simulink model "Pitch_control_v5_test_english"  (R2017b)
settings: Solver=VariableStepAuto  StartTime=0.0  StopTime=60  MaxStep=0.01  RelTol=1e-3
libraries: simulink x2
settings Model: Creator=robo  LastModifiedBy=ad

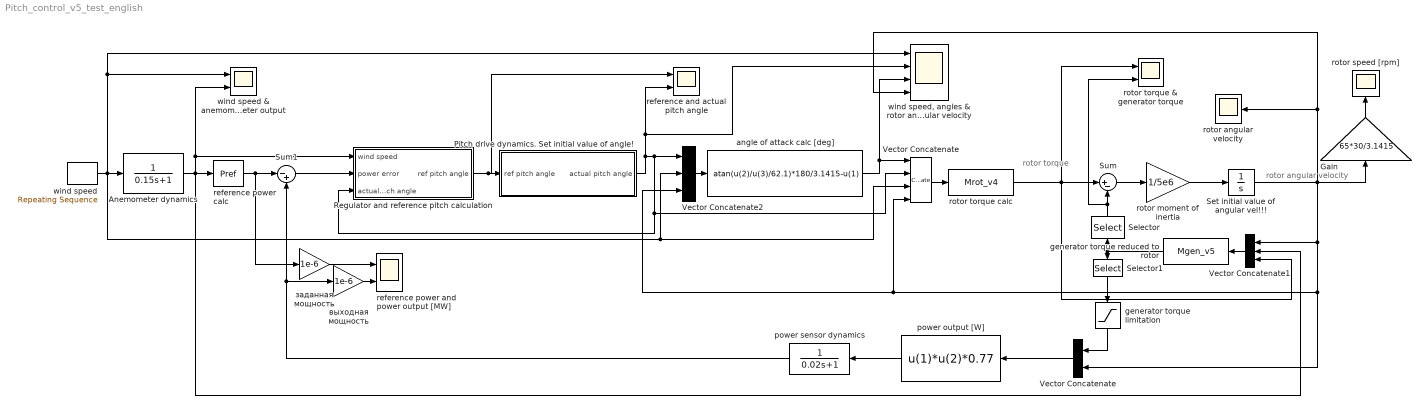
== system Pitch_control_v5_test_english ==
  note: rotor angular velocity
  note: rotor
      | torque
  " rotor moment of inertia " : Gain  Gain=1/5e6
  Anemometer dynamics : TransferFcn  Denominator=[0.15 1]
  Gain : Gain  Gain=65*30/3.1415
  Pitch drive dynamics. Set initial value of angle! : Subsystem
  Regulator and reference pitch calculation : Subsystem
  Selector : Selector  InputPortWidth=2  IndexOptions=Index vector (dialog)  Indices=1  OutputSizes=1
  Selector1 : Selector  InputPortWidth=2  IndexOptions=Index vector (dialog)  Indices=2  OutputSizes=1
  Set initial value of angular vel!!! : Integrator  InitialCondition=10*6/62.1
  Sum : Sum  Inputs=|+-
  Sum1 : Sum  Inputs=|-+
  Vector Concatenate : Concatenate  NumInputs=4
  "Vector Concatenate " : Concatenate
  Vector Concatenate1 : Concatenate  NumInputs=3
  Vector Concatenate2 : Concatenate  NumInputs=3
  angle of attack calc [deg] : Fcn  Expr=atan(u(2)/u(3)/62.1)*180/3.1415-u(1)
  "generator torque reduced to rotor " : S-Function  FunctionName=Mgen_v5  SFunctionDeploymentMode=off  EnableBusSupport=off
  generator torque limitation : Saturate  UpperLimit=5170000  LowerLimit=0
  power output [W] : Fcn  Expr=u(1)*u(2)*0.77
  power sensor dynamics : TransferFcn  Denominator=[0.02 1]
  reference power calc : S-Function  FunctionName=Pref  SFunctionDeploymentMode=off  EnableBusSupport=off
  reference and actual pitch angle : Scope  NumInputPorts=2
  reference power and power output [MW] : Scope  NumInputPorts=2
  rotor speed [rpm] : Scope
  rotor angular velocity : Scope
  rotor torque & generator torque : Scope  NumInputPorts=2
  rotor torque calc : S-Function  FunctionName=Mrot_v4  SFunctionDeploymentMode=off  EnableBusSupport=off
  "wind speed " : simulink/Sources/Repeating Sequence  Description=Входной сигнал по мощности  rep_seq_t=[0 24 28 32 40 44 48 100]  rep_seq_y=[10 10 7 17 17 7 10 10]
  "wind speed & anemometer output " : Scope  NumInputPorts=2
  "wind speed, angles & rotor angular velocity " : Scope  NumInputPorts=4
  выходная мощность : Gain  Gain=1e-6
  заданная мощность : Gain  Gain=1e-6
  wires:
  "wind speed "/1 -> "wind speed, angles & rotor angular velocity "/1, "wind speed & anemometer output "/1, Vector Concatenate/3, Vector Concatenate2/2, Anemometer dynamics/1
  reference power calc/1 -> Sum1/1, заданная мощность/1
  Vector Concatenate2/1 -> angle of attack calc [deg]/1
  Anemometer dynamics/1 -> Vector Concatenate1/2, reference power calc/1, "wind speed & anemometer output "/2, Regulator and reference pitch calculation/1(wind speed)
  Regulator and reference pitch calculation/1(ref pitch angle) -> reference and actual pitch angle/1, Pitch drive dynamics. Set initial value of angle!/1(ref pitch angle)
  Pitch drive dynamics. Set initial value of angle!/1(actual pitch angle) -> reference and actual pitch angle/2, "wind speed, angles & rotor angular velocity "/2, Vector Concatenate/2, Regulator and reference pitch calculation/3(actual pitch angle), Vector Concatenate2/1
  angle of attack calc [deg]/1 -> "wind speed, angles & rotor angular velocity "/3, Vector Concatenate/1
  rotor torque calc/1 -> rotor torque & generator torque/1, Vector Concatenate1/3, Sum/1
  Sum/1 -> " rotor moment of inertia "/1
  " rotor moment of inertia "/1 -> Set initial value of angular vel!!!/1
  "Vector Concatenate "/1 -> power output [W]/1
  power output [W]/1 -> power sensor dynamics/1
  Set initial value of angular vel!!!/1 -> "wind speed, angles & rotor angular velocity "/4, rotor angular velocity/1, Gain/1, Vector Concatenate1/1, "Vector Concatenate "/2, Vector Concatenate2/3, Vector Concatenate/4
  power sensor dynamics/1 -> Sum1/2, выходная мощность/1
  Gain/1 -> rotor speed [rpm]/1
  "generator torque reduced to rotor "/1 -> Selector1/1, Selector/1
  Sum1/1 -> Regulator and reference pitch calculation/2(power error)
  generator torque limitation/1 -> "Vector Concatenate "/1
  Vector Concatenate/1 -> rotor torque calc/1
  Vector Concatenate1/1 -> "generator torque reduced to rotor "/1
  Selector/1 -> rotor torque & generator torque/2, Sum/2
  Selector1/1 -> generator torque limitation/1
  заданная мощность/1 -> reference power and power output [MW]/1
  выходная мощность/1 -> reference power and power output [MW]/2

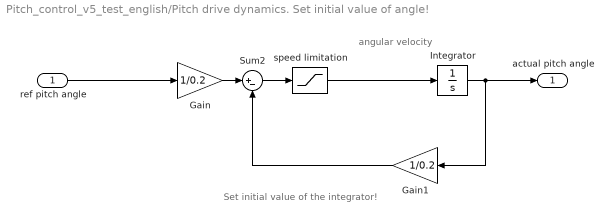
== system Pitch_control_v5_test_english/Pitch drive dynamics. Set initial value of angle! ==
  note: Set initial value of the integrator!
  note: angular
      | velocity
  ref pitch angle : Inport
  Gain : Gain  Gain=1/0.2
  Gain1 : Gain  Gain=1/0.2
  Integrator : Integrator  InitialCondition=-3
  Sum2 : Sum  Inputs=|+-
  speed limitation : Saturate  UpperLimit=12  LowerLimit=-12
  actual pitch angle : Outport
  wires:
  Gain/1 -> Sum2/1
  speed limitation/1 -> Integrator/1
  Sum2/1 -> speed limitation/1
  Gain1/1 -> Sum2/2
  Integrator/1 -> Gain1/1, actual pitch angle/1
  ref pitch angle/1 -> Gain/1

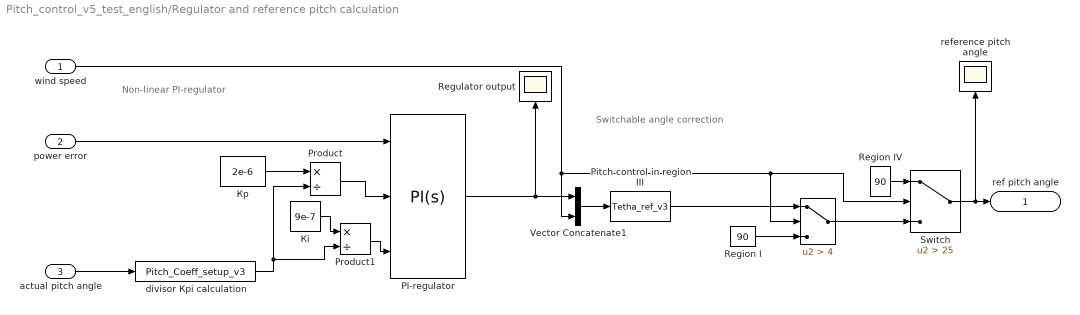
== system Pitch_control_v5_test_english/Regulator and reference pitch calculation ==
  note: Switchable angle correction
  note: Non-linear
      | PI-regulator
  wind speed : Inport
  power error : Inport  Port=2
  actual pitch angle : Inport  Port=3
  " " : Switch  Criteria=u2 > Threshold  Threshold=4
  PI-regulator : simulink/Continuous/PID Controller  Controller=PI  TimeDomain=Continuous-time  SampleTime=-1  IntegratorMethod=Forward Euler  FilterMethod=Forward Euler  Form=Parallel  UseFilter=on  ControllerParametersSource=external  P=1  I=1  D=0  N=100  InitialConditionSource=internal  InitialConditionForIntegrator=0  InitialConditionForFilter=0  ExternalReset=none  LimitOutput=off  UpperSaturationLimit=inf  LowerSaturationLimit=-inf  LinearizeAsGain=on  AntiWindupMode=none  Kb=1  TrackingMode=off  Kt=1  PParamMin=[]  PParamMax=[]  IParamMin=[]  IParamMax=[]  DParamMin=[]  DParamMax=[]  NParamMin=[]  NParamMax=[]  KbParamMin=[]  KbParamMax=[]  KtParamMin=[]  KtParamMax=[]  POutMin=[]  POutMax=[]  IOutMin=[]  IOutMax=[]  DOutMin=[]  DOutMax=[]  NOutMin=[]  NOutMax=[]  KbOutMin=[]  KbOutMax=[]  KtOutMin=[]  KtOutMax=[]  IntegratorOutMin=[]  IntegratorOutMax=[]  FilterOutMin=[]  FilterOutMax=[]  SumOutMin=[]  SumOutMax=[]  SumI1OutMin=[]  SumI1OutMax=[]  SumI2OutMin=[]  SumI2OutMax=[]  SumI3OutMin=[]  SumI3OutMax=[]  SumDOutMin=[]  SumDOutMax=[]  SaturationOutMin=[]  SaturationOutMax=[]  IntegratorContinuousStateAttributes=''  IntegratorStateMustResolveToSignalObject=off  IntegratorRTWStateStorageClass=Auto  FilterContinuousStateAttributes=''  FilterStateMustResolveToSignalObject=off  FilterRTWStateStorageClass=Auto  DifferentiatorICPrevScaledInput=0  DifferentiatorOutMin=[]  DifferentiatorOutMax=[]  InitialConditionSetting=State (most efficient)  FilterDiffOutCoefMin=[]  FilterDiffOutCoefMax=[]  SumDenOutMin=[]  SumDenOutMax=[]  SumNumOutMin=[]  SumNumOutMax=[]  ReciprocalOutMin=[]  ReciprocalOutMax=[]  DivideOutMin=[]  DivideOutMax=[]  TunerSelectOption=Transfer Function Based (PID Tuner App)
  Pitch control in region III : S-Function  FunctionName=Tetha_ref_v3  SFunctionDeploymentMode=off  EnableBusSupport=off
  Product : Product  Inputs=*/
  Product1 : Product  Inputs=*/
  "Region I " : Constant  Value=90
  Region IV : Constant  Value=90
  Regulator output : Scope
  Switch : Switch  Criteria=u2 > Threshold  Threshold=25
  Vector Concatenate1 : Concatenate
  "divisor Кpi calculation " : S-Function  FunctionName=Pitch_Coeff_setup_v3  SFunctionDeploymentMode=off  EnableBusSupport=off
  reference pitch angle : Scope
  Кi : Constant  Value=9e-7
  Кp : Constant  Value=2e-6  VectorParams1D=off
  ref pitch angle : Outport
  wires:
  actual pitch angle/1 -> "divisor Кpi calculation "/1
  Product1/1 -> PI-regulator/3
  "divisor Кpi calculation "/1 -> Product/2, Product1/2
  Кp/1 -> Product/1
  Product/1 -> PI-regulator/2
  Кi/1 -> Product1/1
  power error/1 -> PI-regulator/1
  PI-regulator/1 -> Vector Concatenate1/1, Regulator output/1
  Vector Concatenate1/1 -> Pitch control in region III/1
  " "/1 -> Switch/3
  Region IV/1 -> Switch/1
  Pitch control in region III/1 -> " "/1
  wind speed/1 -> Vector Concatenate1/2, Switch/2, " "/2
  "Region I "/1 -> " "/3
  Switch/1 -> reference pitch angle/1, ref pitch angle/1
